simulink model "Task2_Question1"  (Simulink 8.1)
settings: Solver=FixedStepDiscrete  SolverMode=SingleTasking  StartTime=0.0  StopTime=inf  FixedStep=5e-05  RelTol=1e-3
undefined symbols (not defined in the file or in its folder): dfilt, gcbh, samplefreq, stemdo, upstartman
libraries: dspsigops x6, dsparch4 x4, dspsrcs4 x3, dspmathops x1
(part 2 of 2)

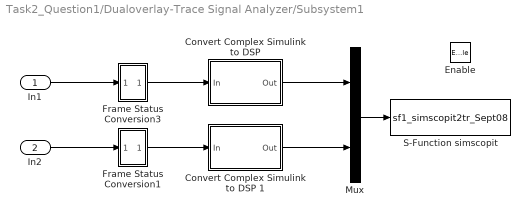
== system Task2_Question1/Dualoverlay-Trace Signal Analyzer/Subsystem1 ==
  In1 : Inport
  In2 : Inport  Port=2
  Enable : EnablePort
  "Convert Complex Simulink to DSP " : Subsystem  mask(Convert Complex Simulink to DSP){}
      mask help: Convert new Simulink complex data type to old DSP Blockset (prior to V3.0) complex data format.
      mask init:
      | [x,y]=cplxico2(1,[]);
      mask Help: web(dspbhelp);
      mask Display:
      | plot(x,y);
      | text(10,50,'Convert\nComplex','horiz','left');
  Convert Complex Simulink to DSP 1 : Subsystem  mask(Convert Complex Simulink to DSP){}
      mask help: Convert new Simulink complex data type to old DSP Blockset (prior to V3.0) complex data format.
      mask init:
      | [x,y]=cplxico2(1,[]);
      mask Help: web(dspbhelp);
      mask Display:
      | plot(x,y);
      | text(10,50,'Convert\nComplex','horiz','left');
  Frame Status Conversion1 : Subsystem  mask(Frame Status Conversion){growRefPort=off, outframe=Sample-based}
      mask prompts: growRefPort "Inherit output frame status from Ref input port"; outframe "Output signal:"
      mask help: Specify the frame status of the output signal.
      mask init:
      | [p, str] = dspblkfrmconv('init');
      mask Help: web(dspbhelp);
      mask Callback growRefPort: dspblkfrmconv
      mask TypeOptions outframe: Frame-based | Sample-based
      mask Display:
      | port_label(p.in1,   p.i1,  p.i1s);
      | port_label(p.in2,   p.i2,  p.i2s);
      | port_label(p.out, p.o1, p.o1s);
      | disp(str)
  Frame Status Conversion3 : Subsystem  mask(Frame Status Conversion){growRefPort=off, outframe=Sample-based}
      mask prompts: growRefPort "Inherit output frame status from Ref input port"; outframe "Output signal:"
      mask help: Specify the frame status of the output signal.
      mask init:
      | [p, str] = dspblkfrmconv('init');
      mask Help: web(dspbhelp);
      mask Callback growRefPort: dspblkfrmconv
      mask TypeOptions outframe: Frame-based | Sample-based
      mask Display:
      | port_label(p.in1,   p.i1,  p.i1s);
      | port_label(p.in2,   p.i2,  p.i2s);
      | port_label(p.out, p.o1, p.o1s);
      | disp(str)
  Mux : Mux  Inputs=2
  S-Function simscopit : S-Function  FunctionName=sf1_simscopit2tr_Sept08  Parameters=name_plot,samplefreq,figpos,stemdo,upstartman,freqtickvec,1  EnableBusSupport=off
  wires:
  Frame Status Conversion1/1(Out) -> Convert Complex Simulink to DSP 1/1(In)
  Frame Status Conversion3/1(Out) -> "Convert Complex Simulink to DSP "/1(In)
  "Convert Complex Simulink to DSP "/1(Out) -> Mux/1
  Convert Complex Simulink to DSP 1/1(Out) -> Mux/2
  In1/1 -> Frame Status Conversion3/1(In1)
  Mux/1 -> S-Function simscopit/1
  In2/1 -> Frame Status Conversion1/1(In1)

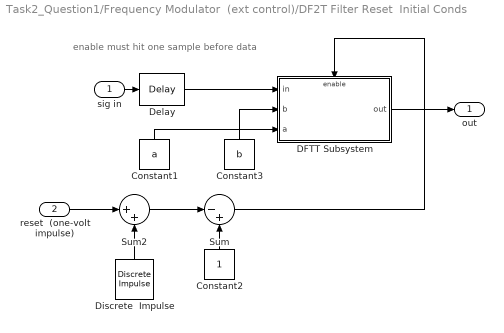
== system Task2_Question1/Frequency Modulator  (ext control)/DF2T Filter Reset  Initial Conds ==
  note: enable must hit one sample
      |  before data
  sig in : Inport
  reset  (one-volt impulse) : Inport  Port=2
  Constant1 : Constant  Value=a
  Constant2 : Constant
  Constant3 : Constant  Value=b
  DFTT Subsystem : Subsystem
  Delay : dspsigops/Delay  InputProcessing=Inherited (this choice will be removed - see release notes)  dly_unit=Samples  delay=1  ic_detail=off  dif_ic_for_ch=off  dif_ic_for_dly=off  ic=0  reset_popup=None
  Discrete  Impulse : dspsrcs4/Discrete  Impulse  Delay=0  SampleTime=ts  FrameSample=1  dataType=double  isSigned=on  wordLen=16  udDataType=sfix(16)  fracBitsMode=Best precision  numFracBits=15  OutDataTypeStr=double  LastOutDataTypeStr=double
  Sum : Sum  Inputs=|-+  SaturateOnIntegerOverflow=on  OutDataTypeStr=Inherit: Same as first input
  Sum2 : Sum  Inputs=|++  SaturateOnIntegerOverflow=on  InputSameDT=on  OutDataTypeStr=Inherit: Same as first input
  out : Outport
  wires:
  Delay/1 -> DFTT Subsystem/1(in)
  sig in/1 -> Delay/1
  DFTT Subsystem/1(out) -> out/1
  Constant2/1 -> Sum/2
  Sum/1 -> DFTT Subsystem/Enable
  Constant1/1 -> DFTT Subsystem/3(a)
  Constant3/1 -> DFTT Subsystem/2(b)
  Discrete  Impulse/1 -> Sum2/2
  reset  (one-volt impulse)/1 -> Sum2/1
  Sum2/1 -> Sum/1

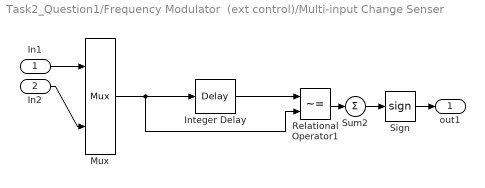
== system Task2_Question1/Frequency Modulator  (ext control)/Multi-input Change Senser ==
  In1 : Inport
  In2 : Inport  Port=2
  Integer Delay : dspsigops/Delay  InputProcessing=Inherited (this choice will be removed - see release notes)  dly_unit=Samples  delay=1  ic_detail=off  dif_ic_for_ch=off  dif_ic_for_dly=off  ic=0  reset_popup=None
  Mux : Mux  Inputs=2
  Relational Operator1 : RelationalOperator  Operator=~=
  Sign : Signum
  Sum2 : Sum  Inputs=1  SaturateOnIntegerOverflow=on
  out1 : Outport
  wires:
  In2/1 -> Mux/2
  Mux/1 -> Relational Operator1/2, Integer Delay/1
  In1/1 -> Mux/1
  Integer Delay/1 -> Relational Operator1/1
  Relational Operator1/1 -> Sum2/1
  Sum2/1 -> Sign/1
  Sign/1 -> out1/1

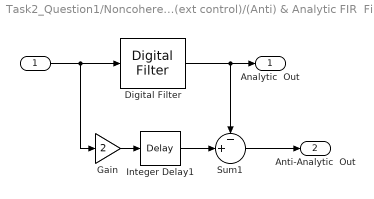
== system Task2_Question1/Noncoherent FM  Demodulator (ext control)/(Anti) & Analytic FIR  Filter (high-grade) ==
  " " : Inport
  Digital Filter : dsparch4/Digital Filter  TypePopup=FIR (all zeros)  IIRFiltStruct=Direct form II transposed  AllPoleFiltStruct=Direct form  FIRFiltStruct=Direct form  CoeffSource=Specify via dialog  NumCoeffs=b  DenCoeffs=[1 0.1]  BiQuadCoeffs=[1 0.3 0.4 1 0.1 0.2]  LatticeCoeffs=[0.2 0.4]  denIgnore=on  FiltPerSampPopup=One filter per frame  IC=icvec  ICnum=0  ICden=0  roundingMode=Floor  overflowMode=off  ScaleValues=1  scaleValueFracLength=14  stageInFracLength=15  stageOutFracLength=15  FilterSource=Specify via dialog  dfiltObjectName=dfilt.dffir([1 2 1])  InputProcessing=Inherited (this choice will be removed - see release notes)
  Gain : Gain  Gain=2  SaturateOnIntegerOverflow=on  OutDataTypeStr=Inherit: Same as input  ParamDataTypeStr=Inherit: Same as input
  Integer Delay1 : dspsigops/Delay  InputProcessing=Inherited (this choice will be removed - see release notes)  dly_unit=Samples  delay=100  ic_detail=off  dif_ic_for_ch=off  dif_ic_for_dly=off  ic=0  reset_popup=None
  Sum1 : Sum  Inputs=-+|  SaturateOnIntegerOverflow=on  InputSameDT=on  OutDataTypeStr=Inherit: Same as first input
  Analytic  Out : Outport  InitialOutput=0
  Anti-Analytic  Out : Outport  Port=2  InitialOutput=0
  wires:
  Gain/1 -> Integer Delay1/1
  Sum1/1 -> Anti-Analytic  Out/1
  Integer Delay1/1 -> Sum1/2
  " "/1 -> Gain/1, Digital Filter/1
  Digital Filter/1 -> Sum1/1, Analytic  Out/1

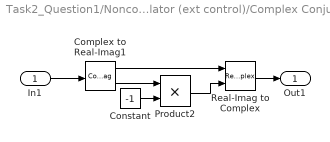
== system Task2_Question1/Noncoherent FM  Demodulator (ext control)/Complex Conjugate ==
  In1 : Inport
  Complex to Real-Imag1 : ComplexToRealImag
  Constant : Constant  Value=-1
  Product2 : Product  SaturateOnIntegerOverflow=on  InputSameDT=on  OutDataTypeStr=Inherit: Same as first input
  Real-Imag to Complex : RealImagToComplex
  Out1 : Outport
  wires:
  Real-Imag to Complex/1 -> Out1/1
  Product2/1 -> Real-Imag to Complex/2
  Constant/1 -> Product2/2
  Complex to Real-Imag1/2 -> Product2/1
  Complex to Real-Imag1/1 -> Real-Imag to Complex/1
  In1/1 -> Complex to Real-Imag1/1

== system Task2_Question1/Noncoherent FM  Demodulator (ext control)/Complexifier ==
  note: a silly thing needed for complex and real coexistence
  In1 : Inport
  Complex to Real-Imag : ComplexToRealImag
  Real-Imag to Complex : RealImagToComplex
  Out1 : Outport
  wires:
  In1/1 -> Complex to Real-Imag/1
  Real-Imag to Complex/1 -> Out1/1
  Complex to Real-Imag/2 -> Real-Imag to Complex/2
  Complex to Real-Imag/1 -> Real-Imag to Complex/1

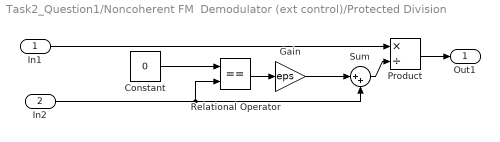
== system Task2_Question1/Noncoherent FM  Demodulator (ext control)/Protected Division ==
  In1 : Inport
  In2 : Inport  Port=2
  Constant : Constant  Value=0
  Gain : Gain  Gain=eps  SaturateOnIntegerOverflow=on  OutDataTypeStr=Inherit: Same as input  ParamDataTypeStr=Inherit: Same as input
  Product : Product  Inputs=*/  SaturateOnIntegerOverflow=on  InputSameDT=on  OutDataTypeStr=Inherit: Same as first input
  Relational Operator : RelationalOperator  Operator===  InputSameDT=on
  Sum : Sum  Inputs=|++  SaturateOnIntegerOverflow=on  InputSameDT=on  OutDataTypeStr=Inherit: Same as first input
  Out1 : Outport  InitialOutput=0
  wires:
  Product/1 -> Out1/1
  Sum/1 -> Product/2
  Gain/1 -> Sum/1
  Relational Operator/1 -> Gain/1
  Constant/1 -> Relational Operator/1
  In2/1 -> Sum/2, Relational Operator/2
  In1/1 -> Product/1

== system Task2_Question1/Noncoherent FM  Demodulator (ext control)/Sliding-Window d.c. Eliminator ==
  note: this acts as a wideband delayor
  In1 : Inport
  N-Point Moving  Averager : Subsystem  mask((non-recursive )N-Point Moving Averager){N=N, normer=off, opcoeffs=off}
      mask prompts: N "N, number of averages:"; normer "Energy-Normalize"; opcoeffs "Output Filter Coefficients"
      mask help:
      | This FIR filter produces an N-point moving average. It is implemented non-recursively, with a transfer function H(z)=(1 +z^-1+...Z^-N)/N.This becomes costly to calculate if N is very large. The user specifies N.
      |
      | In the case of frame-based input, averaging of adjacent sample values is done internal to the frame, or spanning across frame boundaries if N> frame length.
      |
      | The user is able to scale the normal 1/N impulse response values by activating the checkbox "Energy-Normalize", which forces unit impulse response energy.  A second checkbox allows creation of ports for output of the b  coefficient vector.
      mask init:
      | b=ones(1,N)/N;
      | a=1;
      | icvec=0;
      | if(normer);b=b/sqrt(N);end
      | gg=gain(b);
      | mm=max(gg);
      | icvec=0;
      mask Help:
      | This FIR filter produces an N-point moving average. It is implemented non-recursively, with a transfer function H(z)=(1 +z^-1+...Z^-N)/N.This becomes costly to calculate if N is very large. The user specifies N.
      | 
      | In the case of frame-based input, averaging of adjacent sample values is done internal to the frame, or spanning across frame boundaries if N> frame length.
      | 
      | The user is able to scale the normal 1/N impulse response values by activating the checkbox "Energy-Normalize", which forces unit impulse response energy.  A second checkbox allows creation of ports for output of the b  coefficient vector.
      | 
      | Copyright(c) DSP Creations Ltd. 2003-2008.
      mask Callback opcoeffs: constructoutputs(gcb,1)
      mask Display:
      | color('blue')
      | plot([1.1*mm nan gg nan -0.1])
      | color('black')
      | text(0,-.2*mm,[' N= ',num2str(N)])
      | text(0,-.4*mm,[' '])
  Sum : Sum  Inputs=|-+  SaturateOnIntegerOverflow=on  InputSameDT=on  OutDataTypeStr=Inherit: Same as first input
  Out1 : Outport
  wires:
  N-Point Moving  Averager/1(out) -> Sum/1
  In1/1 -> Sum/2, N-Point Moving  Averager/1(" ")
  Sum/1 -> Out1/1

== system Task2_Question1/Periodicize Signal  from Workspace/Fixed Impulse Train ==
  Discrete  Impulse : dspsrcs4/Discrete  Impulse  Delay=0  SampleTime=ts  FrameSample=1  dataType=double  isSigned=on  wordLen=16  udDataType=sfix(16)  fracBitsMode=Best precision  numFracBits=15  OutDataTypeStr=double  LastOutDataTypeStr=double
  Make Input Periodic1 : Subsystem  mask(Periodicizer){N=N}
      mask prompts: N "Period  (in samples)"
      mask help: This block takes any input and (causally) constructs a periodic signal using that. Note that a short period can time-alias the base period.
      mask init:
      | if(isempty(N))
      |     errordlg('ERROR: this value must be set to a positive integer',gcb,'modal')
      | else
      |    maskmaster('passkey_integerize','N',N)
      | end
      mask Help: This auxiliary device produces a (causal) periodic buildup. Normally you let the incoming signal vector  dictate the period (by taking care to set "Period" to be the length of that vector). (See also "Periodicize Signal from Workspace" block).
      mask Display: disp(['Periodicizer\nperiod= ',num2str(N)])
  Out1 : Outport  InitialOutput=0
  wires:
  Make Input Periodic1/1(Out1) -> Out1/1
  Discrete  Impulse/1 -> Make Input Periodic1/1(In1)

== system Task2_Question1/Periodicize Signal  from Workspace/Make Input Periodic ==
  In1 : Inport
  Delay1 : dspsigops/Delay  InputProcessing=Inherited (this choice will be removed - see release notes)  dly_unit=Samples  delay=N  ic_detail=off  dif_ic_for_ch=off  dif_ic_for_dly=off  ic=0  reset_popup=None
  Sum1 : Sum  Inputs=|++  SaturateOnIntegerOverflow=on  InputSameDT=on  OutDataTypeStr=Inherit: Same as first input
  Out1 : Outport  InitialOutput=0
  wires:
  In1/1 -> Sum1/1
  Sum1/1 -> Delay1/1, Out1/1
  Delay1/1 -> Sum1/2

== system Task2_Question1/Dualoverlay-Trace Signal Analyzer/Subsystem/Convert Complex Simulink to DSP  ==
  In : Inport
  Complex to Real-Imag : ComplexToRealImag
  Mux : Mux  Inputs=2
  Out : Outport
  wires:
  Complex to Real-Imag/1 -> Mux/1
  Complex to Real-Imag/2 -> Mux/2
  In/1 -> Complex to Real-Imag/1
  Mux/1 -> Out/1

== system Task2_Question1/Dualoverlay-Trace Signal Analyzer/Subsystem/Convert Complex Simulink to DSP 1 ==
  In : Inport
  Complex to Real-Imag : ComplexToRealImag
  Mux : Mux  Inputs=2
  Out : Outport
  wires:
  Complex to Real-Imag/1 -> Mux/1
  Complex to Real-Imag/2 -> Mux/2
  In/1 -> Complex to Real-Imag/1
  Mux/1 -> Out/1

== system Task2_Question1/Dualoverlay-Trace Signal Analyzer/Subsystem/Frame Status Conversion3 ==
  In1 : Inport
  Frame Status : FrameConversion  OutFrame=Sample-based
  Out : Outport
  wires:
  In1/1 -> Frame Status/1
  Frame Status/1 -> Out/1

== system Task2_Question1/Dualoverlay-Trace Signal Analyzer/Subsystem/Frame Status Conversion4 ==
  In1 : Inport
  Frame Status : FrameConversion  OutFrame=Sample-based
  Out : Outport
  wires:
  Frame Status/1 -> Out/1
  In1/1 -> Frame Status/1

== system Task2_Question1/Dualoverlay-Trace Signal Analyzer/Subsystem1/Convert Complex Simulink to DSP  ==
  In : Inport
  Complex to Real-Imag : ComplexToRealImag
  Mux : Mux  Inputs=2
  Out : Outport
  wires:
  Complex to Real-Imag/1 -> Mux/1
  Complex to Real-Imag/2 -> Mux/2
  In/1 -> Complex to Real-Imag/1
  Mux/1 -> Out/1

== system Task2_Question1/Dualoverlay-Trace Signal Analyzer/Subsystem1/Convert Complex Simulink to DSP 1 ==
  In : Inport
  Complex to Real-Imag : ComplexToRealImag
  Mux : Mux  Inputs=2
  Out : Outport
  wires:
  Complex to Real-Imag/1 -> Mux/1
  Complex to Real-Imag/2 -> Mux/2
  In/1 -> Complex to Real-Imag/1
  Mux/1 -> Out/1

== system Task2_Question1/Dualoverlay-Trace Signal Analyzer/Subsystem1/Frame Status Conversion1 ==
  In1 : Inport
  Frame Status : FrameConversion  OutFrame=Sample-based
  Out : Outport
  wires:
  In1/1 -> Frame Status/1
  Frame Status/1 -> Out/1

== system Task2_Question1/Dualoverlay-Trace Signal Analyzer/Subsystem1/Frame Status Conversion3 ==
  In1 : Inport
  Frame Status : FrameConversion  OutFrame=Sample-based
  Out : Outport
  wires:
  Frame Status/1 -> Out/1
  In1/1 -> Frame Status/1

== system Task2_Question1/Frequency Modulator  (ext control)/DF2T Filter Reset  Initial Conds/DFTT Subsystem ==
  in : Inport
  b : Inport  Port=2
  a : Inport  Port=3
  Enable : EnablePort  StatesWhenEnabling=reset
  Digital Filter : dsparch4/Digital Filter  TypePopup=IIR (poles & zeros)  IIRFiltStruct=Direct form II transposed  AllPoleFiltStruct=Direct form  FIRFiltStruct=Direct form  CoeffSource=Input port(s)  NumCoeffs=[1 2]  DenCoeffs=[1 0.1]  BiQuadCoeffs=[1 0.3 0.4 1 0.1 0.2]  LatticeCoeffs=[0.2 0.4]  denIgnore=on  FiltPerSampPopup=One filter per frame  IC=icvec  ICnum=0  ICden=0  roundingMode=Floor  overflowMode=off  ScaleValues=1  scaleValueFracLength=14  stageInFracLength=15  stageOutFracLength=15  FilterSource=Input port(s)  dfiltObjectName=dfilt.dffir([1 2 1])  InputProcessing=Inherited (this choice will be removed - see release notes)
  out : Outport  OutputWhenDisabled=reset  InitialOutput=Yicvec(1)
  wires:
  in/1 -> Digital Filter/1
  b/1 -> Digital Filter/2
  Digital Filter/1 -> out/1
  a/1 -> Digital Filter/3

== system Task2_Question1/Noncoherent FM  Demodulator (ext control)/Sliding-Window d.c. Eliminator/N-Point Moving  Averager ==
  " " : Inport
  Digital Filter : dsparch4/Digital Filter  TypePopup=FIR (all zeros)  IIRFiltStruct=Direct form II transposed  AllPoleFiltStruct=Direct form  FIRFiltStruct=Direct form  CoeffSource=Input port(s)  NumCoeffs=b  DenCoeffs=[1 0.1]  BiQuadCoeffs=[1 0.3 0.4 1 0.1 0.2]  LatticeCoeffs=[0.2 0.4]  denIgnore=on  FiltPerSampPopup=One filter per frame  IC=icvec  ICnum=0  ICden=0  roundingMode=Floor  overflowMode=off  ScaleValues=1  scaleValueFracLength=14  stageInFracLength=15  stageOutFracLength=15  FilterSource=Input port(s)  dfiltObjectName=dfilt.dffir([1 2 1])  InputProcessing=Inherited (this choice will be removed - see release notes)
  NUM : Constant  Value=b
  out : Outport  InitialOutput=0
  wires:
  NUM/1 -> Digital Filter/2
  Digital Filter/1 -> out/1
  " "/1 -> Digital Filter/1

== system Task2_Question1/Periodicize Signal  from Workspace/Fixed Impulse Train/Make Input Periodic1 ==
  In1 : Inport
  Delay1 : dspsigops/Delay  InputProcessing=Inherited (this choice will be removed - see release notes)  dly_unit=Samples  delay=N  ic_detail=off  dif_ic_for_ch=off  dif_ic_for_dly=off  ic=0  reset_popup=None
  Sum1 : Sum  Inputs=|++  SaturateOnIntegerOverflow=on  InputSameDT=on  OutDataTypeStr=Inherit: Same as first input
  Out1 : Outport  InitialOutput=0
  wires:
  Delay1/1 -> Sum1/2
  Sum1/1 -> Out1/1, Delay1/1
  In1/1 -> Sum1/1
